simulink model "MPC_SCHEME2019B"  (R2023b)
settings: Solver=VariableStepAuto  StartTime=0.0  StopTime=10  FixedStep=0.002  RelTol=1e-3
values from neighbouring files (symbols this model uses):
  A = [0 0 1 0 ... (first row only)    [MPC_RFJ.m]    (also in MPC_integral_RFJ.m; MPC_main_realtime.m; MPCintegral_main_realtime.m)
  A_ob = A - L'*C    [MPC_main_realtime.m]    (also in MPCintegral_main_realtime.m)
  B = eta_m*eta_g*Kc*Kg/Rm*B0    [MPC_RFJ.m]    (also in MPC_integral_RFJ.m; MPC_main_realtime.m; MPCintegral_main_realtime.m)
  B_ob = [B , L']    [MPC_main_realtime.m]    (also in MPCintegral_main_realtime.m)
  C_ob = eye(4)    [MPC_main_realtime.m]    (also in MPCintegral_main_realtime.m)
  N = 5    [MPC_RFJ.m]    (also in MPC_integral_RFJ.m; MPC_main_realtime.m; MPCintegral_main_realtime.m)
  Ts = 0.1    [MPC_RFJ.m]    (also in MPC_integral_RFJ.m; MPC_main_realtime.m; MPCintegral_main_realtime.m)
settings Model: Creator=marco  LastModifiedBy=marco
settings SolverCC: AlgebraicLoopSolver=TrustRegion

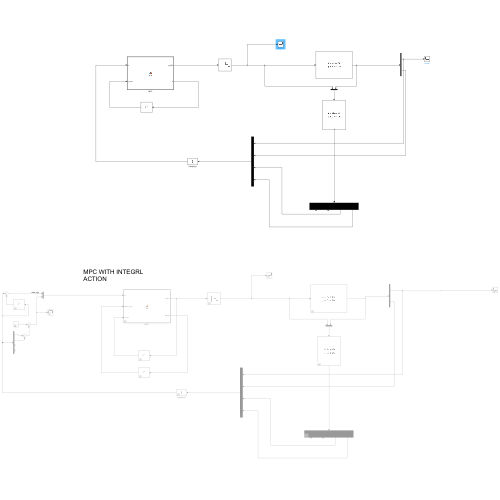
[thumbnail: Simulink's stored preview of the top-level diagram]
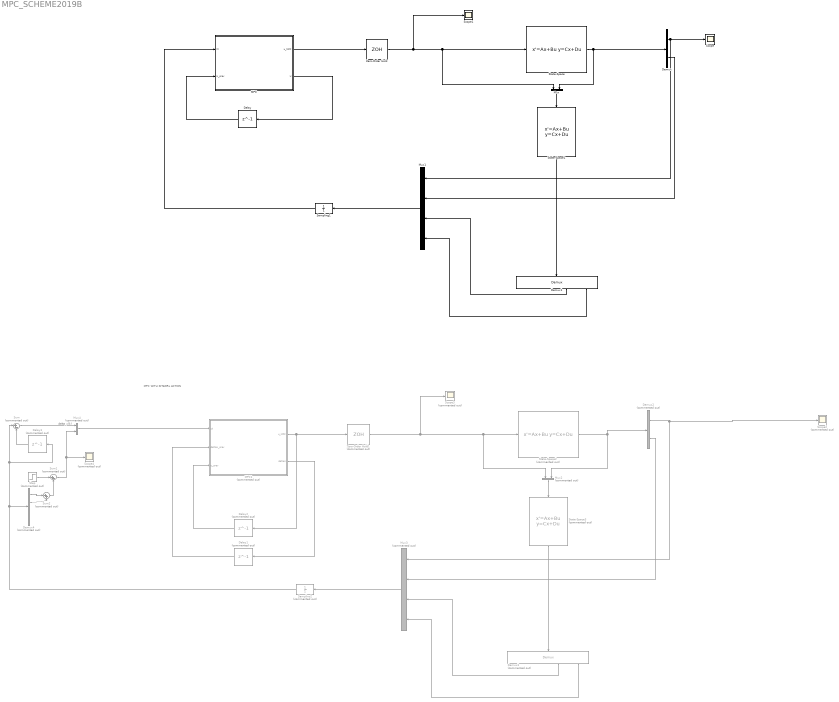
== system MPC_SCHEME2019B ==
  note: delta_x(k)
  note: MPC WITH INTEGRL ACTION
  Delay : Delay  DelayLength=1  InitialCondition=zeros(N,1)  SampleTime=Ts
  Delay1 : Delay  Commented=on  DelayLength=1  InitialCondition=zeros(N,1)  SampleTime=Ts
  Delay2 : Delay  Commented=on  DelayLength=1  InitialCondition=0  SampleTime=Ts
  Delay3 : Delay  Commented=on  DelayLength=1  InitialCondition=zeros(4,1)  SampleTime=Ts
  Demux : Demux  Outputs=2
  Demux1 : Demux
  Demux2 : Demux  Commented=on  Outputs=2
  Demux3 : Demux  Commented=on
  Demux4 : Demux  Commented=on
  MPC : MATLAB Function  TreatAsAtomicUnit=on
  MPC1 : MATLAB Function  Commented=on  TreatAsAtomicUnit=on
  Mux : Mux  Inputs=2
  Mux1 : Mux
  Mux2 : Mux  Commented=on  Inputs=2
  Mux3 : Mux  Commented=on
  Mux4 : Mux  Commented=on  Inputs=2
  Sampling1 : DiscreteTransferFcn  Denominator=[1]  SampleTime=Ts
  Sampling2 : DiscreteTransferFcn  Commented=on  Denominator=[1]  SampleTime=Ts
  Scope : Scope
  Scope1 : Scope
  Scope2 : Scope  Commented=on
  Scope3 : Scope  Commented=on
  Scope4 : Scope  Commented=on
  State-Space : StateSpace  A=A  B=B  C=[1 0 0 0;0 1 0 0]  D=zeros(2,1)  InitialCondition=0
  State-Space1 : StateSpace  A=A_ob  B=B_ob  C=C_ob  D=zeros(4,3)  InitialCondition=0
  State-Space2 : StateSpace  Commented=on  A=A  B=B  C=[1 0 0 0;0 1 0 0]  D=zeros(2,1)  InitialCondition=0
  State-Space3 : StateSpace  Commented=on  A=A_ob  B=B_ob  C=C_ob  D=zeros(4,3)  InitialCondition=0
  Step : Step  Commented=on  After=pi/2  SampleTime=0
  Sum : Sum  Commented=on  Inputs=|+-
  Sum1 : Sum  Commented=on  Inputs=|+-
  Sum2 : Sum  Commented=on  Inputs=|++
  Zero-Order Hold : ZeroOrderHold  SampleTime=Ts
  Zero-Order Hold1 : ZeroOrderHold  Commented=on  SampleTime=Ts
  wires:
  Demux/1 -> Mux1/1, Scope/1
  MPC/2(U) -> Delay/1
  Delay/1 -> MPC/2(U_prev)
  MPC/1(u_MPC) -> Zero-Order Hold/1
  Zero-Order Hold/1 -> Mux/1, State-Space/1, Scope1/1
  State-Space/1 -> Mux/2, Demux/1
  Mux/1 -> State-Space1/1
  State-Space1/1 -> Demux1/1
  Demux/2 -> Mux1/2
  Demux1/3 -> Mux1/3
  Demux1/4 -> Mux1/4
  Mux1/1 -> Sampling1/1
  Sampling1/1 -> MPC/1(zt)
  Demux3/3 -> Mux3/3
  State-Space2/1 -> Demux2/1, Mux2/2
  Mux3/1 -> Sampling2/1
  Mux2/1 -> State-Space3/1
  MPC1/2(deltaU) -> Delay1/1
  Demux3/4 -> Mux3/4
  State-Space3/1 -> Demux3/1
  Demux2/2 -> Mux3/2
  Zero-Order Hold1/1 -> Scope3/1, Mux2/1, State-Space2/1
  Delay1/1 -> MPC1/2(deltaU_prev)
  MPC1/1(u_MPC) -> Delay2/1, Zero-Order Hold1/1
  Demux2/1 -> Mux3/1, Scope2/1
  Delay2/1 -> MPC1/3(u_prev)
  Delay3/1 -> Sum/2
  Mux4/1 -> MPC1/1(zt)
  Sum/1 -> Mux4/1
  Sampling2/1 -> Demux4/1, Delay3/1, Sum/1
  Step/1 -> Sum1/1
  Sum1/1 -> Scope4/1, Mux4/2
  Sum2/1 -> Sum1/2
  Demux4/1 -> Sum2/1
  Demux4/2 -> Sum2/2

== matlab function MPC_SCHEME2019B/MPC1 ==
  data: zt input; u_MPC output; deltaU_prev input; deltaU output; u_prev input
function [u_MPC,deltaU] = fcn(zt,deltaU_prev,u_prev)
%% DISCRETIZED MATRICES (possiamo darle come input dal work space) Ts=0.1 perchè il QP richiede più di due 0.02 secondi per essere risolto nei primi passi
% velocity form matrices

% A=[1.0000    0.4198    0.0428    0.0284         0;
%          0   -0.5120    0.0289    0.0233         0;
%          0   -3.3277    0.4149    0.4152         0;
%          0   -6.3647   -0.2295   -0.5209         0;
%    -1.0000    0.0922   -0.0717   -0.0518    1.0000];
% B= [0 0 63.3952 -63.3952 0]';

C=[0 0 0 0 1];
D=0;

A=[1.0000    0.4198    0.0428    0.0284         0
         0   -0.5120    0.0289    0.0233         0
         0   -3.3277    0.4149    0.4152         0
         0   -6.3647   -0.2295   -0.5209         0
   -1.0000    0.0922   -0.0717   -0.0518    1.0000];

B= [0.0888
   -0.0449
    0.9081
    0.3561
   -0.0439];

%% Signal dimensions
nz     =   5;
nu      =   size(B,2);
ny      =   size(C,1);

%% Prediction horizon and cost function weighting matrices
N       =  5;
Q       =  1;
R       =  1e-2;

%% Inequality constraints
% Input inequalities
Au      =   [eye(nu);-eye(nu)];
bu      =   15*ones(2*nu,1);            % control input rate constrain
nqu     =   size(Au,1);                 % Number of input inequality constraints per stage

% State inequalities
Az     =   [1 0 0 0 0;-1 0 0 0 0];
bz     =   pi/2*ones(2,1); % -180<theta<180
nqz    =   size(Az,1);

%% Reference output and initial state
z0     =   zeros(nz,1);
yref    =   0;

%% Build overall matrices and vectors for QP (note - quadprog solves: min 0.5*x'*H*x + f'*x   subject to:  A*x <= b, Aeq*x = beq)
[Lambda_y,Gamma_y,Lambda_z,Gamma_z]   =   Traj_matrices(N,A,B,C,D);
Qbar                                    =   zeros((N+1)*ny);
Rbar                                    =   zeros(N*nu);
Yref                                    =   zeros((N+1)*ny,1);                              
Aubar                                   =   zeros(N*nqu,N*nu);
bubar                                   =   zeros(N*nqu,1);
Azbar                                  =   zeros((N+1)*nqz,(N+1)*nz); 
bzbar                                  =   zeros((N+1)*nqz,1);

for ind = 1:N+1
    Qbar((ind-1)*ny+1:ind*ny,(ind-1)*ny+1:ind*ny)           =   Q;
    Yref((ind-1)*ny+1:ind*ny,1)                             =   yref;
    Azbar((ind-1)*nqz+1:ind*nqz,(ind-1)*nz+1:ind*nz)   =   Az;
    bzbar((ind-1)*nqz+1:ind*nqz,1)                       =   bz;
end

for ind = 1:N
    Rbar((ind-1)*nu+1:ind*nu,(ind-1)*nu+1:ind*nu)           =   R;
    Aubar((ind-1)*nqu+1:ind*nqu,(ind-1)*nu+1:ind*nu)        =   Au;
    bubar((ind-1)*nqu+1:ind*nqu,1)                          =   bu;
end

Aineq   =   [Aubar;Azbar*Gamma_z];
%Aineq   =   Aubar;
bineq   =   [bubar;bzbar-Azbar*Lambda_z*z0];
%bineq   =   bubar;

% Terminal equality constraint
Aeq     =   Gamma_z(end-nz+1:end,:)-Gamma_z(end-2*nz+1:end-nz,:);
beq     =   -(Lambda_z(end-nz+1:end,:)-Lambda_z(end-2*nz+1:end-nz,:))*z0;

% Cost function
f       =   z0'*Lambda_y'*Qbar*Gamma_y-Yref'*Qbar*Gamma_y;
H       =   (Gamma_y'*Qbar*Gamma_y)+Rbar;
H       =   0.5*(H+H');
u_MPC=0;
bineq                               =   [bubar;bzbar-Azbar*Lambda_z*zt];
beq                                 =   -(Lambda_z(end-nz+1:end,:)-Lambda_z(end-2*nz+1:end-nz,:))*zt;
f                                   =   zt'*Lambda_y'*Qbar*Gamma_y-Yref'*Qbar*Gamma_y;
eml.extrinsic('quadprog');
options = optimoptions('quadprog','Algorithm','active-set'); % comment this row in order to use interior-point algorithm 
deltaU=zeros(N,1);
deltaU                                   =   quadprog(H,f,Aineq,bineq,[],[],[],[],deltaU_prev,options);
u_MPC = u_prev + deltaU(1,1);
deltaU=[deltaU(2:N,1);deltaU(N,1)];

== matlab function MPC_SCHEME2019B/MPC ==
  data: zt input; u_MPC output; U_prev input; U output
function [u_MPC,U] = fcn(zt,U_prev)
Vbar= 15; %maximum voltage
%% DISCRETIZED MATRICES (possiamo darle come input dal work space) Ts=0.1 perchè il QP richiede più di due 0.02 secondi per essere risolto nei primi passi

A=[1.0000    0.4198    0.0428    0.0284;
         0   -0.5120    0.0289    0.0233;
         0   -3.3277    0.4149    0.4152;
         0   -6.3647   -0.2295   -0.5209];
B= [0.0888
   -0.0449
    0.9081
    0.3561];

C=[1 1 0 0];
D=zeros(1,1);

%% Ts 0.5
% A=[1.0000    0.4198    0.0428    0.0284;
%          0   -0.5120    0.0289    0.0233;
%          0   -3.3277    0.4149    0.4152;
%          0   -6.3647   -0.2295   -0.5209];
% 
% B=[0.6829
%     0.0020
%     1.5764
%    -0.0164];
%% Signal dimensions
nz     =   size(A,1);
nu      =   size(B,2);
ny      =   size(C,1);

%% Prediction horizon and cost function weighting matrices
N       =   5;
Q       =   1;
R       =   1e-2;

%% Inequality constraints
% Input inequalities
Au      =   [eye(nu);-eye(nu)];
bu      =   Vbar*ones(2*nu,1);
nqu     =   size(Au,1);                 % Number of input inequality constraints per stage

% State inequalities
Az     =   [1 0 0 0;-1 0 0 0];
bz     =   pi*ones(2,1); % -180<theta<180
nqz    =   size(Az,1);

%% Reference output and initial state
z0     =   zeros(nz,1);
yref    =   pi/2*ones(ny,1);

%% Build overall matrices and vectors for QP (note - quadprog solves: min 0.5*x'*H*x + f'*x   subject to:  A*x <= b, Aeq*x = beq)
[Lambda_y,Gamma_y,Lambda_z,Gamma_z]   =   Traj_matrices(N,A,B,C,D);
Qbar                                    =   zeros((N+1)*ny);
Rbar                                    =   zeros(N*nu);
Yref                                    =   zeros((N+1)*ny,1);                              
Aubar                                   =   zeros(N*nqu,N*nu);
bubar                                   =   zeros(N*nqu,1);
Azbar                                  =   zeros((N+1)*nqz,(N+1)*nz); 
bzbar                                  =   zeros((N+1)*nqz,1);

for ind = 1:N+1
    Qbar((ind-1)*ny+1:ind*ny,(ind-1)*ny+1:ind*ny)           =   Q;
    Yref((ind-1)*ny+1:ind*ny,1)                             =   yref;
    Azbar((ind-1)*nqz+1:ind*nqz,(ind-1)*nz+1:ind*nz)   =   Az;
    bzbar((ind-1)*nqz+1:ind*nqz,1)                       =   bz;
end

for ind = 1:N
    Rbar((ind-1)*nu+1:ind*nu,(ind-1)*nu+1:ind*nu)           =   R;
    Aubar((ind-1)*nqu+1:ind*nqu,(ind-1)*nu+1:ind*nu)        =   Au;
    bubar((ind-1)*nqu+1:ind*nqu,1)                          =   bu;
end

Aineq   =   [Aubar;Azbar*Gamma_z];
bineq   =   [bubar;bzbar-Azbar*Lambda_z*z0];

% Terminal equality constraint
Aeq     =   Gamma_z(end-nz+1:end,:)-Gamma_z(end-2*nz+1:end-nz,:);
beq     =   -(Lambda_z(end-nz+1:end,:)-Lambda_z(end-2*nz+1:end-nz,:))*z0;

% Cost function
f       =   z0'*Lambda_y'*Qbar*Gamma_y-Yref'*Qbar*Gamma_y;
H       =   (Gamma_y'*Qbar*Gamma_y)+Rbar;
H       =   0.5*(H+H');
u_MPC=0;
bineq                               =   [bubar;bzbar-Azbar*Lambda_z*zt];
beq                                 =   -(Lambda_z(end-nz+1:end,:)-Lambda_z(end-2*nz+1:end-nz,:))*zt;
f                                   =   zt'*Lambda_y'*Qbar*Gamma_y-Yref'*Qbar*Gamma_y;
% eml.extrinsic('quadprog');
options = optimoptions('quadprog','Algorithm','active-set'); % comment this row in order to use interior-point algorithm 
U=zeros(N,1);
U                                   =   quadprog(H,f,Aineq,bineq,Aeq,beq,[],[],U_prev,options);
u_MPC =   U(1,nu);
U=[U(2:N,1);U(N,1)];
